simulink model "user_cmd_io"  (R2021a)
settings: Solver=FixedStepAuto  StartTime=0.0  StopTime=100.0  RelTol=1e-3
undefined symbols (not defined in the file): f
libraries: dspnetwork x9, slrealtimeiplib x9, slrealtimeutilitieslib x7, simulink x5, instrumentlib x1
settings Model: SimulationMode=accelerator  Creator=Ruixuan  LastModifiedBy=Charles
settings SolverCC: ConcurrentTasks=on  PositivePriorityOrder=on  AutoInsertRateTranBlk=on  InsertRTBMode=Never (minimum delay)
settings OptimizationCC: BlockReduction=off  DefaultParameterBehavior=Inlined  OptimizeBlockIOStorage=off
settings DebuggingCC: TasksWithSamePriorityMsg=none
settings HardwareCC: ProdBitPerLong=64  ProdLongLongMode=on  ProdHWDeviceType=Intel->x86-64 (Linux 64)
settings ModelReferenceCC: ModelReferenceNumInstancesAllowed=Single
settings RTWCC: Description=Simulink Real-Time  SystemTargetFile=slrealtime.tlc  TemplateMakefile=slrealtime_default_tmf  Toolchain=Simulink Real-Time Toolchain  BuildConfiguration=Faster Runs  CodeExecutionProfiling=on  TargetLang=C++

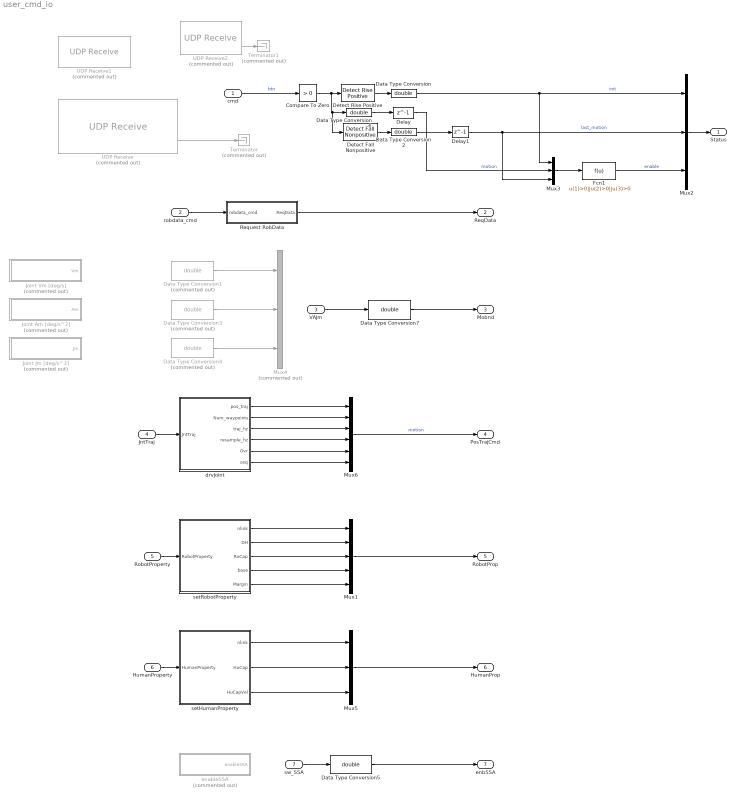
== system user_cmd_io ==
  cmd : Inport
  robdata_cmd : Inport  Port=2
  VAJm : Inport  Port=3
  JntTraj : Inport  Port=4
  RobotProperty : Inport  Port=5
  HumanProperty : Inport  Port=6
  sw_SSA : Inport  Port=7
  Compare To Zero : simulink/Logic and Bit Operations/Compare To Zero  relop=>  OutDataTypeStr=boolean
  Data Type Conversion{,2,5..7} (5 alike) : DataTypeConversion  OutDataTypeStr=double
  Data Type Conversion1 : DataTypeConversion  Commented=on  OutDataTypeStr=double
  Data Type Conversion3 : DataTypeConversion  Commented=on  OutDataTypeStr=double
  Data Type Conversion4 : DataTypeConversion  Commented=on  OutDataTypeStr=double
  Delay : Delay  DelayLength=1  InitialCondition=0
  Delay1 : Delay  DelayLength=1  InitialCondition=0
  Detect Fall Nonpositive : simulink/Logic and Bit Operations/Detect Fall Nonpositive  vinit=1  OutDataTypeStr=boolean
      settings: SourceProductBaseCode=SL
  Detect Rise Positive : simulink/Logic and Bit Operations/Detect Rise Positive  vinit=0  OutDataTypeStr=boolean
  Fcn1 : Fcn  Expr=u(1)>0||u(2)>0||u(3)>0
  Joint Am [deg/s^2] : Subsystem  Commented=on  mask(CartPosTrjLimit){}
  Joint Jm [deg/s^3] : Subsystem  Commented=on  mask(CartPosTrjLimit){}
  Joint Vm [deg/s] : Subsystem  Commented=on  mask(CartPosTrjLimit){}
  Mux1 : Mux  Inputs=[1,40,70,3,1]
  Mux2 : Mux  Inputs=3
  Mux3 : Mux  Inputs=3
  Mux4 : Mux  Commented=on  Inputs=3
  Mux5 : Mux  Inputs=[1,70,60]
  Mux6 : Mux  Inputs=[11250,1,1,1,1,1]
  Request RobData : Subsystem  mask(CartPosTrjLimit){}
  Terminator : Terminator  Commented=on
  Terminator1 : Terminator  Commented=on
  UDP Receive : slrealtimeiplib/UDP Receive  Commented=on  useHostTargetConn=on  ipAddress=10.10.10.15  localPort=8001  rcvWidth=1  rcvFmAny=on  fmAddress=192.168.7.2  sampleTime=Ts
      settings: SourceProductBaseCode=XP
  UDP Receive1 : instrumentlib/UDP Receive  Commented=on  Host=localhost  Port=9090  LocalPort=8888  EnablePortSharing=off  GetLatestData=off  DataSize=[1 1]  DataType=uint8  ASCIIFormatting=%f,  Terminator=LF  ByteOrder=BigEndian  EnableBlockingMode=on  Timeout=10  SampleTime=0.01  LocalAddress=0.0.0.0
  UDP Receive2 : dspnetwork/UDP Receive  Commented=on  localURL='0.0.0.0'  localPort=8001  remoteURL='0.0.0.0'  remotePort=-1  recvBufferSize=8192  dims=1  signalDatatype=uint8  isComplex=off  isVarSize=off  showBlockingTime=on  blockingTime=inf  sampletime=Ts  blockPlatform=HOST
  drvJoint : Subsystem  mask(DesiredPoseUserInput){}
  enableSSA : Subsystem  Commented=on  mask(CartPosTrjLimit){}
  setHumanProperty : Subsystem  mask(DesiredPoseUserInput){}
  setRobotProperty : Subsystem  mask(DesiredPoseUserInput){}
  Status : Outport  VectorParamsAs1DForOutWhenUnconnected=off
  ReqData : Outport  Port=2  VectorParamsAs1DForOutWhenUnconnected=off
  Mobnd : Outport  Port=3  VectorParamsAs1DForOutWhenUnconnected=off
  PosTrajCmd : Outport  Port=4  VectorParamsAs1DForOutWhenUnconnected=off
  RobotProp : Outport  Port=5  VectorParamsAs1DForOutWhenUnconnected=off
  HumanProp : Outport  Port=6  VectorParamsAs1DForOutWhenUnconnected=off
  enbSSA : Outport  Port=7  VectorParamsAs1DForOutWhenUnconnected=off
  wires:
  Compare To Zero/1 -> Detect Fall Nonpositive/1, Data Type Conversion6/1, Detect Rise Positive/1
  Fcn1/1 -> Mux2/3  "enable"
  Mux2/1 -> Status/1
  Data Type Conversion2/1 -> Delay1/1
  Detect Rise Positive/1 -> Data Type Conversion/1
  Delay/1 -> Mux3/2  "motion"
  Detect Fall Nonpositive/1 -> Data Type Conversion2/1
  UDP Receive/2 -> Terminator/1
  cmd/1 -> Compare To Zero/1  "btn"
  Mux3/1 -> Fcn1/1
  Delay1/1 -> Mux3/3, Mux2/2  "last_motion"
  Data Type Conversion3/1 -> Mux4/2
  Data Type Conversion/1 -> Mux3/1, Mux2/1  "init"
  Data Type Conversion6/1 -> Delay/1
  Data Type Conversion4/1 -> Mux4/3
  Data Type Conversion7/1 -> Mobnd/1
  Request RobData/1(ReqData) -> ReqData/1
  Mux1/1 -> RobotProp/1
  setRobotProperty/5(Margin) -> Mux1/5
  setRobotProperty/4(base) -> Mux1/4
  setRobotProperty/3(RoCap) -> Mux1/3
  setRobotProperty/2(DH) -> Mux1/2
  setRobotProperty/1(nlink) -> Mux1/1
  setHumanProperty/1(nlink) -> Mux5/1
  setHumanProperty/2(HuCap) -> Mux5/2
  Mux5/1 -> HumanProp/1
  Data Type Conversion5/1 -> enbSSA/1
  setHumanProperty/3(HuCapVel) -> Mux5/3
  UDP Receive2/2 -> Terminator1/1
  robdata_cmd/1 -> Request RobData/1(robdata_cmd)
  Data Type Conversion1/1 -> Mux4/1
  drvJoint/1(pos_traj) -> Mux6/1
  drvJoint/2(Num_waypoints) -> Mux6/2
  drvJoint/3(traj_hz) -> Mux6/3
  drvJoint/4(resample_hz) -> Mux6/4
  drvJoint/5(Ovr) -> Mux6/5
  drvJoint/6(seq) -> Mux6/6
  Mux6/1 -> PosTrajCmd/1  "motion"
  JntTraj/1 -> drvJoint/1(JntTraj)
  RobotProperty/1 -> setRobotProperty/1(RobotProperty)
  HumanProperty/1 -> setHumanProperty/1(HumanProperty)
  sw_SSA/1 -> Data Type Conversion5/1
  VAJm/1 -> Data Type Conversion7/1

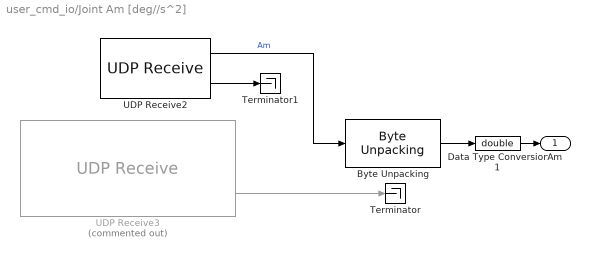
== system user_cmd_io/Joint Am [deg//s^2] ==
  "Byte Unpacking " : slrealtimeutilitieslib/Byte Unpacking  MaskUnpackedDataTypes={'single'}  MaskUnpackedDataSizes={[6]}  MaskAlignment=1
      settings: SourceProductBaseCode=XP
  Data Type Conversion1 : DataTypeConversion  OutDataTypeStr=double
  Terminator : Terminator
  Terminator1 : Terminator
  UDP Receive2 : dspnetwork/UDP Receive  localURL='0.0.0.0'  localPort=8004  remoteURL='0.0.0.0'  remotePort=-1  recvBufferSize=8192  dims=6  signalDatatype=single  isComplex=off  isVarSize=off  showBlockingTime=on  blockingTime=inf  sampletime=Ts  blockPlatform=HOST
  UDP Receive3 : slrealtimeiplib/UDP Receive  Commented=on  useHostTargetConn=on  ipAddress=10.10.10.15  localPort=8004  rcvWidth=24  rcvFmAny=on  fmAddress=192.168.7.2  sampleTime=Ts
      settings: SourceProductBaseCode=XP
  Am : Outport  VectorParamsAs1DForOutWhenUnconnected=off
  wires:
  UDP Receive3/2 -> Terminator/1
  UDP Receive2/1 -> "Byte Unpacking "/1  "Am"
  "Byte Unpacking "/1 -> Data Type Conversion1/1
  Data Type Conversion1/1 -> Am/1
  UDP Receive2/2 -> Terminator1/1

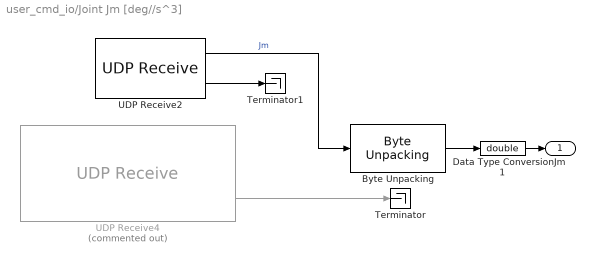
== system user_cmd_io/Joint Jm [deg//s^3] ==
  "Byte Unpacking " : slrealtimeutilitieslib/Byte Unpacking  MaskUnpackedDataTypes={'single'}  MaskUnpackedDataSizes={[6]}  MaskAlignment=1
      settings: SourceProductBaseCode=XP
  Data Type Conversion1 : DataTypeConversion  OutDataTypeStr=double
  Terminator : Terminator
  Terminator1 : Terminator
  UDP Receive2 : dspnetwork/UDP Receive  localURL='0.0.0.0'  localPort=8005  remoteURL='0.0.0.0'  remotePort=-1  recvBufferSize=8192  dims=6  signalDatatype=single  isComplex=off  isVarSize=off  showBlockingTime=on  blockingTime=inf  sampletime=Ts  blockPlatform=HOST
  UDP Receive4 : slrealtimeiplib/UDP Receive  Commented=on  useHostTargetConn=on  ipAddress=10.10.10.15  localPort=8005  rcvWidth=24  rcvFmAny=on  fmAddress=192.168.7.2  sampleTime=Ts
      settings: SourceProductBaseCode=XP
  Jm : Outport  VectorParamsAs1DForOutWhenUnconnected=off
  wires:
  UDP Receive4/2 -> Terminator/1
  UDP Receive2/1 -> "Byte Unpacking "/1  "Jm"
  "Byte Unpacking "/1 -> Data Type Conversion1/1
  Data Type Conversion1/1 -> Jm/1
  UDP Receive2/2 -> Terminator1/1

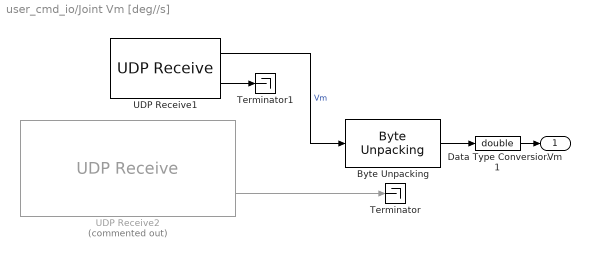
== system user_cmd_io/Joint Vm [deg//s] ==
  "Byte Unpacking " : slrealtimeutilitieslib/Byte Unpacking  MaskUnpackedDataTypes={'single'}  MaskUnpackedDataSizes={[6]}  MaskAlignment=1
      settings: SourceProductBaseCode=XP
  Data Type Conversion1 : DataTypeConversion  OutDataTypeStr=double
  Terminator : Terminator
  Terminator1 : Terminator
  UDP Receive1 : dspnetwork/UDP Receive  localURL='0.0.0.0'  localPort=8003  remoteURL='0.0.0.0'  remotePort=-1  recvBufferSize=8192  dims=6  signalDatatype=single  isComplex=off  isVarSize=off  showBlockingTime=on  blockingTime=inf  sampletime=Ts  blockPlatform=HOST
  UDP Receive2 : slrealtimeiplib/UDP Receive  Commented=on  useHostTargetConn=on  ipAddress=10.10.10.15  localPort=8003  rcvWidth=24  rcvFmAny=on  fmAddress=192.168.7.2  sampleTime=Ts
      settings: SourceProductBaseCode=XP
  Vm : Outport  VectorParamsAs1DForOutWhenUnconnected=off
  wires:
  UDP Receive2/2 -> Terminator/1
  UDP Receive1/1 -> "Byte Unpacking "/1  "Vm"
  "Byte Unpacking "/1 -> Data Type Conversion1/1
  Data Type Conversion1/1 -> Vm/1
  UDP Receive1/2 -> Terminator1/1

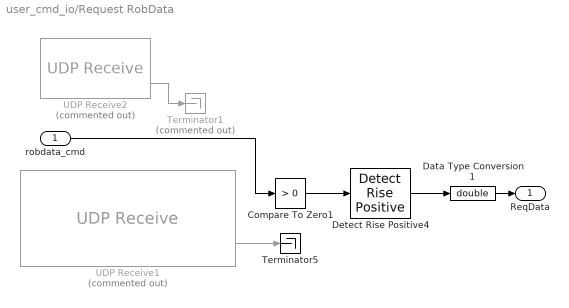
== system user_cmd_io/Request RobData ==
  robdata_cmd : Inport
  Compare To Zero1 : simulink/Logic and Bit Operations/Compare To Zero  relop=>  OutDataTypeStr=boolean
  Data Type Conversion1 : DataTypeConversion  OutDataTypeStr=double
  Detect Rise Positive4 : simulink/Logic and Bit Operations/Detect Rise Positive  vinit=0  OutDataTypeStr=boolean
  Terminator1 : Terminator  Commented=on
  Terminator5 : Terminator
  UDP Receive1 : slrealtimeiplib/UDP Receive  Commented=on  useHostTargetConn=on  ipAddress=10.10.10.15  localPort=8106  rcvWidth=1  rcvFmAny=on  fmAddress=0.0.0.0  sampleTime=Ts
      settings: SourceProductBaseCode=XP
  UDP Receive2 : dspnetwork/UDP Receive  Commented=on  localURL='0.0.0.0'  localPort=8106  remoteURL='0.0.0.0'  remotePort=-1  recvBufferSize=8192  dims=1  signalDatatype=uint8  isComplex=off  isVarSize=off  showBlockingTime=on  blockingTime=inf  sampletime=Ts  blockPlatform=HOST
  ReqData : Outport  VectorParamsAs1DForOutWhenUnconnected=off
  wires:
  Data Type Conversion1/1 -> ReqData/1
  UDP Receive1/2 -> Terminator5/1
  Compare To Zero1/1 -> Detect Rise Positive4/1
  robdata_cmd/1 -> Compare To Zero1/1
  Detect Rise Positive4/1 -> Data Type Conversion1/1
  UDP Receive2/2 -> Terminator1/1

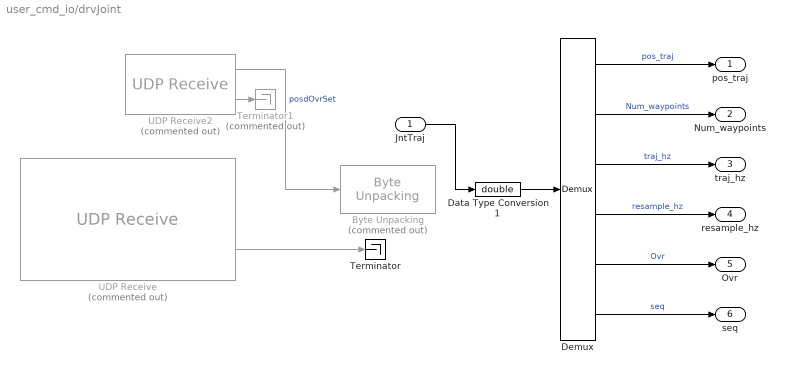
== system user_cmd_io/drvJoint ==
  JntTraj : Inport
  "Byte Unpacking " : slrealtimeutilitieslib/Byte Unpacking  Commented=on  MaskUnpackedDataTypes={'single'}  MaskUnpackedDataSizes={[11255]}  MaskAlignment=1
      settings: SourceProductBaseCode=XP
  Data Type Conversion1 : DataTypeConversion  OutDataTypeStr=double
  Demux : Demux  Outputs=[11250,1,1,1,1,1]
      settings: DisplayOption=none
  Terminator : Terminator
  Terminator1 : Terminator  Commented=on
  UDP Receive : slrealtimeiplib/UDP Receive  Commented=on  useHostTargetConn=on  ipAddress=10.10.10.15  localPort=8104  rcvWidth=45020  rcvFmAny=on  fmAddress=192.168.7.2  sampleTime=Ts
      settings: SourceProductBaseCode=XP
  UDP Receive2 : dspnetwork/UDP Receive  Commented=on  localURL='0.0.0.0'  localPort=8104  remoteURL='0.0.0.0'  remotePort=-1  recvBufferSize=11255  dims=11255  signalDatatype=single  isComplex=off  isVarSize=off  showBlockingTime=on  blockingTime=inf  sampletime=Ts  blockPlatform=HOST
  pos_traj : Outport  VectorParamsAs1DForOutWhenUnconnected=off
  Num_waypoints : Outport  Port=2  VectorParamsAs1DForOutWhenUnconnected=off
  traj_hz : Outport  Port=3  VectorParamsAs1DForOutWhenUnconnected=off
  resample_hz : Outport  Port=4  VectorParamsAs1DForOutWhenUnconnected=off
  Ovr : Outport  Port=5  VectorParamsAs1DForOutWhenUnconnected=off
  seq : Outport  Port=6  VectorParamsAs1DForOutWhenUnconnected=off
  wires:
  UDP Receive2/1 -> "Byte Unpacking "/1  "posdOvrSet"
  JntTraj/1 -> Data Type Conversion1/1
  UDP Receive/2 -> Terminator/1
  Data Type Conversion1/1 -> Demux/1
  Demux/1 -> pos_traj/1  "pos_traj"
  Demux/5 -> Ovr/1  "Ovr"
  Demux/6 -> seq/1  "seq"
  Demux/2 -> Num_waypoints/1  "Num_waypoints"
  Demux/3 -> traj_hz/1  "traj_hz"
  Demux/4 -> resample_hz/1  "resample_hz"
  UDP Receive2/2 -> Terminator1/1

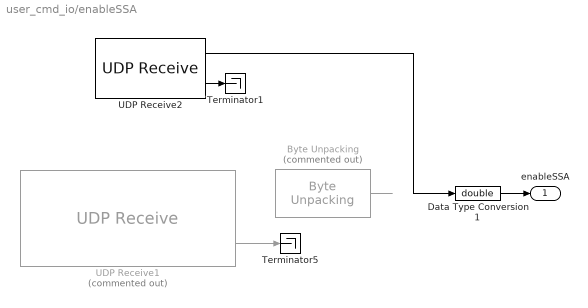
== system user_cmd_io/enableSSA ==
  "Byte Unpacking " : slrealtimeutilitieslib/Byte Unpacking  Commented=on  MaskUnpackedDataTypes={'single'}  MaskUnpackedDataSizes={[1]}  MaskAlignment=1
      settings: SourceProductBaseCode=XP
  Data Type Conversion1 : DataTypeConversion  OutDataTypeStr=double
  Terminator1 : Terminator
  Terminator5 : Terminator
  UDP Receive1 : slrealtimeiplib/UDP Receive  Commented=on  useHostTargetConn=on  ipAddress=10.10.10.15  localPort=8105  rcvWidth=4  rcvFmAny=on  fmAddress=0.0.0.0  sampleTime=Ts
      settings: SourceProductBaseCode=XP
  UDP Receive2 : dspnetwork/UDP Receive  localURL='0.0.0.0'  localPort=8105  remoteURL='0.0.0.0'  remotePort=-1  recvBufferSize=8192  dims=1  signalDatatype=uint8  isComplex=off  isVarSize=off  showBlockingTime=on  blockingTime=inf  sampletime=Ts  blockPlatform=HOST
  enableSSA : Outport  VectorParamsAs1DForOutWhenUnconnected=off
  wires:
  Data Type Conversion1/1 -> enableSSA/1
  UDP Receive1/2 -> Terminator5/1
  UDP Receive2/1 -> Data Type Conversion1/1
  "Byte Unpacking "/1 -> ?
  UDP Receive2/2 -> Terminator1/1

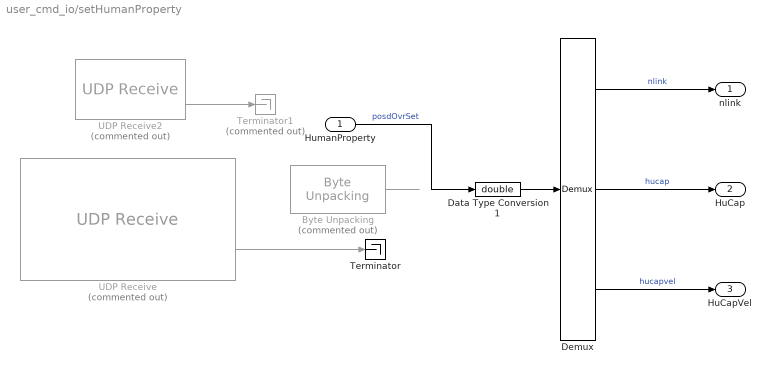
== system user_cmd_io/setHumanProperty ==
  HumanProperty : Inport
  "Byte Unpacking " : slrealtimeutilitieslib/Byte Unpacking  Commented=on  MaskUnpackedDataTypes={'single'}  MaskUnpackedDataSizes={[131]}  MaskAlignment=1
      settings: SourceProductBaseCode=XP
  Data Type Conversion1 : DataTypeConversion  OutDataTypeStr=double
  Demux : Demux  Outputs=[1,70,60]
      settings: DisplayOption=none
  Terminator : Terminator
  Terminator1 : Terminator  Commented=on
  UDP Receive : slrealtimeiplib/UDP Receive  Commented=on  useHostTargetConn=on  ipAddress=10.10.10.15  localPort=8108  rcvWidth=524  rcvFmAny=on  fmAddress=192.168.7.2  sampleTime=Ts
      settings: SourceProductBaseCode=XP
  UDP Receive2 : dspnetwork/UDP Receive  Commented=on  localURL='0.0.0.0'  localPort=8108  remoteURL='0.0.0.0'  remotePort=-1  recvBufferSize=8192  dims=131  signalDatatype=single  isComplex=off  isVarSize=off  showBlockingTime=on  blockingTime=inf  sampletime=Ts  blockPlatform=HOST
  nlink : Outport  VectorParamsAs1DForOutWhenUnconnected=off
  HuCap : Outport  Port=2  VectorParamsAs1DForOutWhenUnconnected=off
  HuCapVel : Outport  Port=3  VectorParamsAs1DForOutWhenUnconnected=off
  wires:
  HumanProperty/1 -> Data Type Conversion1/1  "posdOvrSet"
  "Byte Unpacking "/1 -> ?
  UDP Receive/2 -> Terminator/1
  Data Type Conversion1/1 -> Demux/1
  Demux/1 -> nlink/1  "nlink"
  Demux/2 -> HuCap/1  "hucap"
  Demux/3 -> HuCapVel/1  "hucapvel"
  UDP Receive2/2 -> Terminator1/1

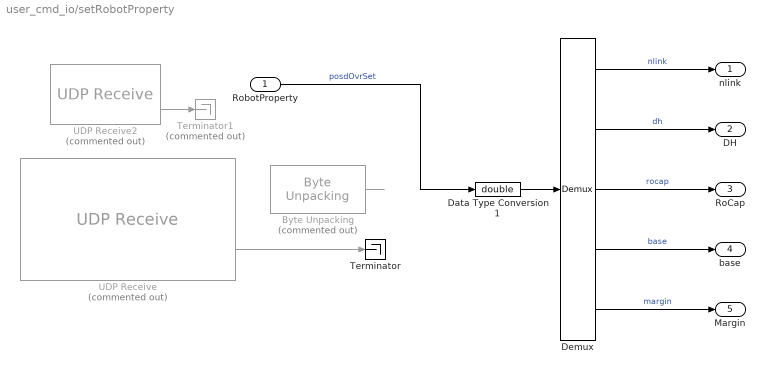
== system user_cmd_io/setRobotProperty ==
  RobotProperty : Inport
  "Byte Unpacking " : slrealtimeutilitieslib/Byte Unpacking  Commented=on  MaskUnpackedDataTypes={'single'}  MaskUnpackedDataSizes={[115]}  MaskAlignment=1
      settings: SourceProductBaseCode=XP
  Data Type Conversion1 : DataTypeConversion  OutDataTypeStr=double
  Demux : Demux  Outputs=[1,40,70,3,1]
      settings: DisplayOption=none
  Terminator : Terminator
  Terminator1 : Terminator  Commented=on
  UDP Receive : slrealtimeiplib/UDP Receive  Commented=on  useHostTargetConn=on  ipAddress=10.10.10.15  localPort=8107  rcvWidth=460  rcvFmAny=on  fmAddress=192.168.7.2  sampleTime=Ts
      settings: SourceProductBaseCode=XP
  UDP Receive2 : dspnetwork/UDP Receive  Commented=on  localURL='0.0.0.0'  localPort=8107  remoteURL='0.0.0.0'  remotePort=-1  recvBufferSize=115  dims=115  signalDatatype=single  isComplex=off  isVarSize=off  showBlockingTime=on  blockingTime=inf  sampletime=Ts  blockPlatform=HOST
  nlink : Outport  VectorParamsAs1DForOutWhenUnconnected=off
  DH : Outport  Port=2  VectorParamsAs1DForOutWhenUnconnected=off
  RoCap : Outport  Port=3  VectorParamsAs1DForOutWhenUnconnected=off
  base : Outport  Port=4  VectorParamsAs1DForOutWhenUnconnected=off
  Margin : Outport  Port=5  VectorParamsAs1DForOutWhenUnconnected=off
  wires:
  RobotProperty/1 -> Data Type Conversion1/1  "posdOvrSet"
  "Byte Unpacking "/1 -> ?
  UDP Receive/2 -> Terminator/1
  Data Type Conversion1/1 -> Demux/1
  Demux/1 -> nlink/1  "nlink"
  Demux/5 -> Margin/1  "margin"
  Demux/2 -> DH/1  "dh"
  Demux/3 -> RoCap/1  "rocap"
  Demux/4 -> base/1  "base"
  UDP Receive2/2 -> Terminator1/1
